simulink model "Demo_PreScanCarSim3D_ExtFMU_cs"  (Simulink 8.6)
settings: Solver=ode5  SolverMode=SingleTasking  StartTime=0.0  StopTime=68  FixedStep=1/1000  RelTol=1e-3
PreLoadFcn:
  | mbxruntime.callbacks.PreLoadFcn(bdroot);
  | check_NUTS_defined;
  | 
  | assignin('base',['model_closed_' bdroot],false);
PostLoadFcn:
  | mbxruntime.callbacks.PostLoadFcn(bdroot);
InitFcn:
  | mbxruntime.callbacks.InitFcn(bdroot);
StartFcn:
  | mbxruntime.callbacks.StartFcn(bdroot);
StopFcn:
  | mbxruntime.callbacks.StopFcn(bdroot);
undefined symbols (not defined in the file): DiscIntNeverNeededParam, mbxruntime, tabledata, warningInitialVelocity, x0, x_ini_VRML, y_ini_VRML, z_ini_VRML
libraries: PreScanSimulinkLibrary x15, simulink_extras x8, simulink x5, PreScanCarSimLibrary x1
(part 4 of 11)

== system Demo_PreScanCarSim3D_ExtFMU_cs/Audi_A8_1/ENABLED/VISUWheelsCarSim_Mux ==
  StateWheels : Inport
  Bus Selector : BusSelector  OutputSignals=PreScanBUS_VehicleDynamics.Wheel.Position.Linear.Pos_FL_Wheel_CoorSys_V[x;y;z][m],PreScanBUS_VehicleDynamics.Wheel.Position.Angualr.Rot_FL_Wheel_CoorSys_V[x;y;z][deg].Angle_Camber_FL_Wheel_CoorSys_V[deg],PreScanBUS_VehicleDynamics.Wheel.Position.Angualr.Rot_FL_Wheel_CoorSys_V[x;y;z][deg].Angle_Rot_FL_Wheel[deg],PreScanBUS_VehicleDynamics.Wheel.Position.Angualr.Rot_FL_Wheel_CoorSys_V[x;y;z][deg].Angle_Toe_FL_Wheel_CoorSys_V[deg],PreScanBUS_VehicleDynamics.Wheel.Position.Linear.Pos_FR_Wheel_CoorSys_V[x;y;z][m],PreScanBUS_VehicleDynamics.Wheel.Position.Angualr.Rot_FR_Wheel_CoorSys_V[x;y;z][deg].Angle_Camber_FR_Wheel_CoorSys_V[deg],PreScanBUS_VehicleDynamics.Wheel.Position.Angualr.Rot_FR_Wheel_CoorSys_V[x;y;z][deg].Angle_Rot_FR_Wheel[deg],PreScanBUS_VehicleDynamics.Wheel.Position.Angualr.Rot_FR_Wheel_CoorSys_V[x;y;z][deg].Angle_Toe_FR_Wheel_CoorSys_V[deg],PreScanBUS_VehicleDynamics.Wheel.Position.Linear.Pos_RL_Wheel_CoorSys_V[x;y;z][m],PreScanBUS_VehicleDynamics.Wheel.Position.Angualr.Rot_RL_Wheel_CoorSys_V[x;y;z][deg].Angle_Camber_RL_Wheel_CoorSys_V[deg],PreScanBUS_VehicleDynamics.Wheel.Position.Angualr.Rot_RL_Wheel_CoorSys_V[x;y;z][deg].Angle_Rot_RL_Wheel[deg],PreScanBUS_VehicleDynamics.Wheel.Position.Angualr.Rot_RL_Wheel_CoorSys_V[x;y;z][deg].Angle_Toe_RL_Wheel_CoorSys_V[deg],PreScanBUS_VehicleDynamics.Wheel.Position.Linear.Pos_RR_Wheel_CoorSys_V[x;y;z][m],PreScanBUS_VehicleDynamics.Wheel.Position.Angualr.Rot_RR_Wheel_CoorSys_V[x;y;z][deg].Angle_Camber_RR_Wheel_CoorSys_V[deg],PreScanBUS_VehicleDynamics.Wheel.Position.Angualr.Rot_RR_Wheel_CoorSys_V[x;y;z][deg].Angle_Rot_RR_Wheel[deg],PreScanBUS_VehicleDynamics.Wheel.Position.Angualr.Rot_RR_Wheel_CoorSys_V[x;y;z][deg].Angle_Toe_RR_Wheel_CoorSys_V[deg]
  Demux{,1..3} (4 alike) : Demux  Outputs=3
  Mux{,1..4,6..8} (8 alike) : Mux  Inputs=3
  Mux5 : Mux  Inputs=[3 3 3 3 3 3 3 3]
  Wheels : Outport
  wires:
  Bus Selector/16 -> Mux3/3  "<Angle_Toe_RR_Wheel_CoorSys_V[deg]>"
  Bus Selector/15 -> Mux3/2  "<Angle_Rot_RR_Wheel[deg]>"
  Bus Selector/14 -> Mux3/1  "<Angle_Camber_RR_Wheel_CoorSys_V[deg]>"
  Bus Selector/13 -> Demux3/1  "<Pos_RR_Wheel_CoorSys_V[x;y;z][m]>"
  Demux3/3 -> Mux8/3
  Demux3/2 -> Mux8/2
  Demux3/1 -> Mux8/1
  Bus Selector/12 -> Mux2/3  "<Angle_Toe_RL_Wheel_CoorSys_V[deg]>"
  Bus Selector/11 -> Mux2/2  "<Angle_Rot_RL_Wheel[deg]>"
  Bus Selector/10 -> Mux2/1  "<Angle_Camber_RL_Wheel_CoorSys_V[deg]>"
  Bus Selector/9 -> Demux2/1  "<Pos_RL_Wheel_CoorSys_V[x;y;z][m]>"
  Demux2/3 -> Mux7/3
  Demux2/2 -> Mux7/2
  Demux2/1 -> Mux7/1
  Bus Selector/8 -> Mux1/3  "<Angle_Toe_FR_Wheel_CoorSys_V[deg]>"
  Bus Selector/7 -> Mux1/2  "<Angle_Rot_FR_Wheel[deg]>"
  Bus Selector/6 -> Mux1/1  "<Angle_Camber_FR_Wheel_CoorSys_V[deg]>"
  Bus Selector/5 -> Demux1/1  "<Pos_FR_Wheel_CoorSys_V[x;y;z][m]>"
  Demux1/3 -> Mux6/3
  Demux1/2 -> Mux6/2
  Demux1/1 -> Mux6/1
  Bus Selector/4 -> Mux/3  "<Angle_Toe_FL_Wheel_CoorSys_V[deg]>"
  Bus Selector/3 -> Mux/2  "<Angle_Rot_FL_Wheel[deg]>"
  Bus Selector/2 -> Mux/1  "<Angle_Camber_FL_Wheel_CoorSys_V[deg]>"
  Demux/3 -> Mux4/3
  Demux/2 -> Mux4/2
  Demux/1 -> Mux4/1
  Bus Selector/1 -> Demux/1  "<Pos_FL_Wheel_CoorSys_V[x;y;z][m]>"
  StateWheels/1 -> Bus Selector/1
  Mux2/1 -> Mux5/6  "xyz rotation RL [deg]"
  Mux3/1 -> Mux5/8  "xyz rotation RR [deg]"
  Mux/1 -> Mux5/2  "xyz rotation FL [deg]"
  Mux1/1 -> Mux5/4  "xyz rotation FR [deg]"
  Mux5/1 -> Wheels/1
  Mux4/1 -> Mux5/1  "xyz displacement FL [m]"
  Mux6/1 -> Mux5/3  "xyz displacement FR [m]"
  Mux8/1 -> Mux5/7  "xyz displacement RR [m]"
  Mux7/1 -> Mux5/5  "xyz displacement RL [m]"

== system Demo_PreScanCarSim3D_ExtFMU_cs/Box_1/DISABLED/GND1 ==
  GND_AccelerationX : Constant  Value=0
  GND_AccelerationY : Constant  Value=0
  GND_AccelerationZ : Constant  Value=0
  GND_AngularVelocityPitch : Constant  Value=0
  GND_AngularVelocityRoll : Constant  Value=0
  GND_AngularVelocityYaw : Constant  Value=0
  GND_OrientationPitch : Constant  Value=0
  GND_OrientationRoll : Constant  Value=0
  GND_OrientationYaw : Constant  Value=0
  GND_PositionX : Constant  Value=0
  GND_PositionY : Constant  Value=0
  GND_PositionZ : Constant  Value=0
  GND_VelocityX : Constant  Value=0
  GND_VelocityY : Constant  Value=0
  GND_VelocityZ : Constant  Value=0
  buscreator : BusCreator  Inputs=15  OutDataTypeStr=Bus: PRESCAN_STATEACTUATORDATA  NonVirtualBus=on
  bus : Outport  OutDataTypeStr=Bus: PRESCAN_STATEACTUATORDATA
  wires:
  GND_PositionX/1 -> buscreator/1  "PositionX"
  GND_PositionY/1 -> buscreator/2  "PositionY"
  GND_PositionZ/1 -> buscreator/3  "PositionZ"
  GND_VelocityX/1 -> buscreator/4  "VelocityX"
  GND_VelocityY/1 -> buscreator/5  "VelocityY"
  GND_VelocityZ/1 -> buscreator/6  "VelocityZ"
  GND_AccelerationX/1 -> buscreator/7  "AccelerationX"
  GND_AccelerationY/1 -> buscreator/8  "AccelerationY"
  GND_AccelerationZ/1 -> buscreator/9  "AccelerationZ"
  GND_OrientationRoll/1 -> buscreator/10  "OrientationRoll"
  GND_OrientationPitch/1 -> buscreator/11  "OrientationPitch"
  GND_OrientationYaw/1 -> buscreator/12  "OrientationYaw"
  GND_AngularVelocityRoll/1 -> buscreator/13  "AngularVelocityRoll"
  GND_AngularVelocityPitch/1 -> buscreator/14  "AngularVelocityPitch"
  GND_AngularVelocityYaw/1 -> buscreator/15  "AngularVelocityYaw"
  buscreator/1 -> bus/1

== system Demo_PreScanCarSim3D_ExtFMU_cs/Box_1/ENABLED/Dynamics_Empty ==
  note: For state mode 'Dynamic' positions
      | are not taken into account, as they
      | are computed by integrating velocity.
      | Click annotation for Help.
  Ground_{1..9} (9 alike) : Ground
  MuxState : Subsystem  Tag=mux/State  mask(Empty Dynamics State Block){positioningmode=on, TimeStep=50/1000}
      mask prompts: positioningmode "Positioning Mode"; TimeStep "Auto Assigned: Time Step [s]"
      mask help:
      | Build the state of an actor based on user input.
      | The user can either use positioning mode or dynamics mode.
      | - When using positioning mode the position and orientation of the actor are set directly based on the input. Expected input is relative to the initial position and orientation of the actor. It's also possible to specify the velocity of the actor, though this input isn't used, only passed on.
      | - When using dynamics mode the position input is ignored. Expected input is velocity and orientation. The velocity is relative the current orientation of the actor, while orientation is relative to its initial orientation. The position of the actor is calculated based on the velocity and orientation given.
      settings: DeleteFcn=PreScanBlockDeleteFcn;
  State : Outport  Tag=outport/StateOutport  SampleTime=50/1000
  wires:
  MuxState/1(state) -> State/1
  Ground_1/1 -> MuxState/1(x [m])
  Ground_2/1 -> MuxState/2(y [m])
  Ground_3/1 -> MuxState/3(z [m])
  Ground_4/1 -> MuxState/4(dx [m/s])
  Ground_5/1 -> MuxState/5(dy [m/s])
  Ground_6/1 -> MuxState/6(dz [m/s])
  Ground_7/1 -> MuxState/7(R [rad])
  Ground_8/1 -> MuxState/8(P [rad])
  Ground_9/1 -> MuxState/9(Y [rad])

== system Demo_PreScanCarSim3D_ExtFMU_cs/Box_1/ENABLED/SELF_Demux ==
  SELF : Inport  OutDataTypeStr=Bus: PRESCAN_SELFSENSORDATA
  Bus Selector : BusSelector  OutputSignals=PositionX,PositionY,PositionZ,OrientationRoll,OrientationPitch,OrientationYaw,Velocity,Yaw_rate,Lat,Long,Alt
  Demux2 : Demux  Outputs=3
  Gain : Gain  Gain=180/pi
  Gain1 : Gain  Gain=180/pi
  Vector Concatenate1 : Concatenate  NumInputs=3
  compas converter : Subsystem
  x [m] : Outport
  y [m] : Outport  Port=2
  z [m] : Outport  Port=3
  rotx [deg] : Outport  Port=4
  roty [deg] : Outport  Port=5
  rotz [deg] : Outport  Port=6
  GPS lat [deg] : Outport  Port=7
  GPS long [deg] : Outport  Port=8
  GPS alt [m] : Outport  Port=9
  velocity [m/s] : Outport  Port=10
  heading [deg] : Outport  Port=11
  yaw rate [deg/s] : Outport  Port=12
  wires:
  Bus Selector/11 -> GPS alt [m]/1  "<Alt>"
  Bus Selector/10 -> GPS long [deg]/1  "<Long>"
  Bus Selector/9 -> GPS lat [deg]/1  "<Lat>"
  Bus Selector/8 -> Gain1/1  "<Yaw_rate>"
  Bus Selector/7 -> velocity [m/s]/1  "<Velocity>"
  Bus Selector/6 -> compas converter/1(rotz [rad]), Vector Concatenate1/3  "<OrientationYaw>"
  Bus Selector/5 -> Vector Concatenate1/2  "<OrientationPitch>"
  Bus Selector/4 -> Vector Concatenate1/1  "<OrientationRoll>"
  Vector Concatenate1/1 -> Gain/1
  Bus Selector/3 -> z [m]/1  "<PositionZ>"
  Bus Selector/2 -> y [m]/1  "<PositionY>"
  Bus Selector/1 -> x [m]/1  "<PositionX>"
  SELF/1 -> Bus Selector/1
  Gain/1 -> Demux2/1
  Demux2/1 -> rotx [deg]/1
  Demux2/2 -> roty [deg]/1
  Demux2/3 -> rotz [deg]/1
  compas converter/1(heading [deg]) -> heading [deg]/1
  Gain1/1 -> yaw rate [deg/s]/1

== system Demo_PreScanCarSim3D_ExtFMU_cs/Box_1/ENABLED/STATE_Box_1 ==
  State : Inport  SampleTime=TimeStep
  Bus Creator : BusCreator  Inputs=15  OutDataTypeStr=Bus: PRESCAN_STATEACTUATORDATA  NonVirtualBus=on
  Demux : Demux  Outputs=15
  iniBODYAngles wrtVEH [rad] : Constant  Value=[Roll0 Pitch0 0]  SampleTime=TimeStep
  iniVEHAngles wrtGLOB [rad] : Constant  Value=[0 0 Yaw0]  SampleTime=TimeStep
  iniVEHposition wrtGLOB [m] : Constant  Value=[x0 y0 z0]  SampleTime=TimeStep
  state2FullState : PreScanSimulinkLibrary/state2FullState  SystemSampleTime=-1
  StateBus : Outport  OutDataTypeStr=Bus: PRESCAN_STATEACTUATORDATA
  wires:
  Bus Creator/1 -> StateBus/1
  State/1 -> state2FullState/1
  state2FullState/1 -> Demux/1
  iniVEHposition wrtGLOB [m]/1 -> state2FullState/2
  iniBODYAngles wrtVEH [rad]/1 -> state2FullState/3
  iniVEHAngles wrtGLOB [rad]/1 -> state2FullState/4
  Demux/1 -> Bus Creator/1  "PositionX"
  Demux/2 -> Bus Creator/2  "PositionY"
  Demux/3 -> Bus Creator/3  "PositionZ"
  Demux/4 -> Bus Creator/4  "VelocityX"
  Demux/5 -> Bus Creator/5  "VelocityY"
  Demux/6 -> Bus Creator/6  "VelocityZ"
  Demux/7 -> Bus Creator/7  "AccelerationX"
  Demux/8 -> Bus Creator/8  "AccelerationY"
  Demux/9 -> Bus Creator/9  "AccelerationZ"
  Demux/10 -> Bus Creator/10  "OrientationRoll"
  Demux/11 -> Bus Creator/11  "OrientationPitch"
  Demux/12 -> Bus Creator/12  "OrientationYaw"
  Demux/13 -> Bus Creator/13  "AngularVelocityRoll"
  Demux/14 -> Bus Creator/14  "AngularVelocityPitch"
  Demux/15 -> Bus Creator/15  "AngularVelocityYaw"

== system Demo_PreScanCarSim3D_ExtFMU_cs/Box_2/DISABLED/GND1 ==
  GND_AccelerationX : Constant  Value=0
  GND_AccelerationY : Constant  Value=0
  GND_AccelerationZ : Constant  Value=0
  GND_AngularVelocityPitch : Constant  Value=0
  GND_AngularVelocityRoll : Constant  Value=0
  GND_AngularVelocityYaw : Constant  Value=0
  GND_OrientationPitch : Constant  Value=0
  GND_OrientationRoll : Constant  Value=0
  GND_OrientationYaw : Constant  Value=0
  GND_PositionX : Constant  Value=0
  GND_PositionY : Constant  Value=0
  GND_PositionZ : Constant  Value=0
  GND_VelocityX : Constant  Value=0
  GND_VelocityY : Constant  Value=0
  GND_VelocityZ : Constant  Value=0
  buscreator : BusCreator  Inputs=15  OutDataTypeStr=Bus: PRESCAN_STATEACTUATORDATA  NonVirtualBus=on
  bus : Outport  OutDataTypeStr=Bus: PRESCAN_STATEACTUATORDATA
  wires:
  GND_PositionX/1 -> buscreator/1  "PositionX"
  GND_PositionY/1 -> buscreator/2  "PositionY"
  GND_PositionZ/1 -> buscreator/3  "PositionZ"
  GND_VelocityX/1 -> buscreator/4  "VelocityX"
  GND_VelocityY/1 -> buscreator/5  "VelocityY"
  GND_VelocityZ/1 -> buscreator/6  "VelocityZ"
  GND_AccelerationX/1 -> buscreator/7  "AccelerationX"
  GND_AccelerationY/1 -> buscreator/8  "AccelerationY"
  GND_AccelerationZ/1 -> buscreator/9  "AccelerationZ"
  GND_OrientationRoll/1 -> buscreator/10  "OrientationRoll"
  GND_OrientationPitch/1 -> buscreator/11  "OrientationPitch"
  GND_OrientationYaw/1 -> buscreator/12  "OrientationYaw"
  GND_AngularVelocityRoll/1 -> buscreator/13  "AngularVelocityRoll"
  GND_AngularVelocityPitch/1 -> buscreator/14  "AngularVelocityPitch"
  GND_AngularVelocityYaw/1 -> buscreator/15  "AngularVelocityYaw"
  buscreator/1 -> bus/1

== system Demo_PreScanCarSim3D_ExtFMU_cs/Box_2/ENABLED/Dynamics_Empty ==
  note: For state mode 'Dynamic' positions
      | are not taken into account, as they
      | are computed by integrating velocity.
      | Click annotation for Help.
  Ground_{1..9} (9 alike) : Ground
  MuxState : Subsystem  Tag=mux/State  mask(Empty Dynamics State Block){positioningmode=on, TimeStep=50/1000}
      mask prompts: positioningmode "Positioning Mode"; TimeStep "Auto Assigned: Time Step [s]"
      mask help:
      | Build the state of an actor based on user input.
      | The user can either use positioning mode or dynamics mode.
      | - When using positioning mode the position and orientation of the actor are set directly based on the input. Expected input is relative to the initial position and orientation of the actor. It's also possible to specify the velocity of the actor, though this input isn't used, only passed on.
      | - When using dynamics mode the position input is ignored. Expected input is velocity and orientation. The velocity is relative the current orientation of the actor, while orientation is relative to its initial orientation. The position of the actor is calculated based on the velocity and orientation given.
      settings: DeleteFcn=PreScanBlockDeleteFcn;
  State : Outport  Tag=outport/StateOutport  SampleTime=50/1000
  wires:
  MuxState/1(state) -> State/1
  Ground_1/1 -> MuxState/1(x [m])
  Ground_2/1 -> MuxState/2(y [m])
  Ground_3/1 -> MuxState/3(z [m])
  Ground_4/1 -> MuxState/4(dx [m/s])
  Ground_5/1 -> MuxState/5(dy [m/s])
  Ground_6/1 -> MuxState/6(dz [m/s])
  Ground_7/1 -> MuxState/7(R [rad])
  Ground_8/1 -> MuxState/8(P [rad])
  Ground_9/1 -> MuxState/9(Y [rad])

== system Demo_PreScanCarSim3D_ExtFMU_cs/Box_2/ENABLED/SELF_Demux ==
  SELF : Inport  OutDataTypeStr=Bus: PRESCAN_SELFSENSORDATA
  Bus Selector : BusSelector  OutputSignals=PositionX,PositionY,PositionZ,OrientationRoll,OrientationPitch,OrientationYaw,Velocity,Yaw_rate,Lat,Long,Alt
  Demux2 : Demux  Outputs=3
  Gain : Gain  Gain=180/pi
  Gain1 : Gain  Gain=180/pi
  Vector Concatenate1 : Concatenate  NumInputs=3
  compas converter : Subsystem
  x [m] : Outport
  y [m] : Outport  Port=2
  z [m] : Outport  Port=3
  rotx [deg] : Outport  Port=4
  roty [deg] : Outport  Port=5
  rotz [deg] : Outport  Port=6
  GPS lat [deg] : Outport  Port=7
  GPS long [deg] : Outport  Port=8
  GPS alt [m] : Outport  Port=9
  velocity [m/s] : Outport  Port=10
  heading [deg] : Outport  Port=11
  yaw rate [deg/s] : Outport  Port=12
  wires:
  Bus Selector/11 -> GPS alt [m]/1  "<Alt>"
  Bus Selector/10 -> GPS long [deg]/1  "<Long>"
  Bus Selector/9 -> GPS lat [deg]/1  "<Lat>"
  Bus Selector/8 -> Gain1/1  "<Yaw_rate>"
  Bus Selector/7 -> velocity [m/s]/1  "<Velocity>"
  Bus Selector/6 -> compas converter/1(rotz [rad]), Vector Concatenate1/3  "<OrientationYaw>"
  Bus Selector/5 -> Vector Concatenate1/2  "<OrientationPitch>"
  Bus Selector/4 -> Vector Concatenate1/1  "<OrientationRoll>"
  Vector Concatenate1/1 -> Gain/1
  Bus Selector/3 -> z [m]/1  "<PositionZ>"
  Bus Selector/2 -> y [m]/1  "<PositionY>"
  Bus Selector/1 -> x [m]/1  "<PositionX>"
  SELF/1 -> Bus Selector/1
  Gain/1 -> Demux2/1
  Demux2/1 -> rotx [deg]/1
  Demux2/2 -> roty [deg]/1
  Demux2/3 -> rotz [deg]/1
  compas converter/1(heading [deg]) -> heading [deg]/1
  Gain1/1 -> yaw rate [deg/s]/1

== system Demo_PreScanCarSim3D_ExtFMU_cs/Box_2/ENABLED/STATE_Box_2 ==
  State : Inport  SampleTime=TimeStep
  Bus Creator : BusCreator  Inputs=15  OutDataTypeStr=Bus: PRESCAN_STATEACTUATORDATA  NonVirtualBus=on
  Demux : Demux  Outputs=15
  iniBODYAngles wrtVEH [rad] : Constant  Value=[Roll0 Pitch0 0]  SampleTime=TimeStep
  iniVEHAngles wrtGLOB [rad] : Constant  Value=[0 0 Yaw0]  SampleTime=TimeStep
  iniVEHposition wrtGLOB [m] : Constant  Value=[x0 y0 z0]  SampleTime=TimeStep
  state2FullState : PreScanSimulinkLibrary/state2FullState  SystemSampleTime=-1
  StateBus : Outport  OutDataTypeStr=Bus: PRESCAN_STATEACTUATORDATA
  wires:
  Bus Creator/1 -> StateBus/1
  State/1 -> state2FullState/1
  state2FullState/1 -> Demux/1
  iniVEHposition wrtGLOB [m]/1 -> state2FullState/2
  iniBODYAngles wrtVEH [rad]/1 -> state2FullState/3
  iniVEHAngles wrtGLOB [rad]/1 -> state2FullState/4
  Demux/1 -> Bus Creator/1  "PositionX"
  Demux/2 -> Bus Creator/2  "PositionY"
  Demux/3 -> Bus Creator/3  "PositionZ"
  Demux/4 -> Bus Creator/4  "VelocityX"
  Demux/5 -> Bus Creator/5  "VelocityY"
  Demux/6 -> Bus Creator/6  "VelocityZ"
  Demux/7 -> Bus Creator/7  "AccelerationX"
  Demux/8 -> Bus Creator/8  "AccelerationY"
  Demux/9 -> Bus Creator/9  "AccelerationZ"
  Demux/10 -> Bus Creator/10  "OrientationRoll"
  Demux/11 -> Bus Creator/11  "OrientationPitch"
  Demux/12 -> Bus Creator/12  "OrientationYaw"
  Demux/13 -> Bus Creator/13  "AngularVelocityRoll"
  Demux/14 -> Bus Creator/14  "AngularVelocityPitch"
  Demux/15 -> Bus Creator/15  "AngularVelocityYaw"

== system Demo_PreScanCarSim3D_ExtFMU_cs/Box_3/DISABLED/GND1 ==
  GND_AccelerationX : Constant  Value=0
  GND_AccelerationY : Constant  Value=0
  GND_AccelerationZ : Constant  Value=0
  GND_AngularVelocityPitch : Constant  Value=0
  GND_AngularVelocityRoll : Constant  Value=0
  GND_AngularVelocityYaw : Constant  Value=0
  GND_OrientationPitch : Constant  Value=0
  GND_OrientationRoll : Constant  Value=0
  GND_OrientationYaw : Constant  Value=0
  GND_PositionX : Constant  Value=0
  GND_PositionY : Constant  Value=0
  GND_PositionZ : Constant  Value=0
  GND_VelocityX : Constant  Value=0
  GND_VelocityY : Constant  Value=0
  GND_VelocityZ : Constant  Value=0
  buscreator : BusCreator  Inputs=15  OutDataTypeStr=Bus: PRESCAN_STATEACTUATORDATA  NonVirtualBus=on
  bus : Outport  OutDataTypeStr=Bus: PRESCAN_STATEACTUATORDATA
  wires:
  GND_PositionX/1 -> buscreator/1  "PositionX"
  GND_PositionY/1 -> buscreator/2  "PositionY"
  GND_PositionZ/1 -> buscreator/3  "PositionZ"
  GND_VelocityX/1 -> buscreator/4  "VelocityX"
  GND_VelocityY/1 -> buscreator/5  "VelocityY"
  GND_VelocityZ/1 -> buscreator/6  "VelocityZ"
  GND_AccelerationX/1 -> buscreator/7  "AccelerationX"
  GND_AccelerationY/1 -> buscreator/8  "AccelerationY"
  GND_AccelerationZ/1 -> buscreator/9  "AccelerationZ"
  GND_OrientationRoll/1 -> buscreator/10  "OrientationRoll"
  GND_OrientationPitch/1 -> buscreator/11  "OrientationPitch"
  GND_OrientationYaw/1 -> buscreator/12  "OrientationYaw"
  GND_AngularVelocityRoll/1 -> buscreator/13  "AngularVelocityRoll"
  GND_AngularVelocityPitch/1 -> buscreator/14  "AngularVelocityPitch"
  GND_AngularVelocityYaw/1 -> buscreator/15  "AngularVelocityYaw"
  buscreator/1 -> bus/1

== system Demo_PreScanCarSim3D_ExtFMU_cs/Box_3/ENABLED/Dynamics_Empty ==
  note: For state mode 'Dynamic' positions
      | are not taken into account, as they
      | are computed by integrating velocity.
      | Click annotation for Help.
  Ground_{1..9} (9 alike) : Ground
  MuxState : Subsystem  Tag=mux/State  mask(Empty Dynamics State Block){positioningmode=on, TimeStep=50/1000}
      mask prompts: positioningmode "Positioning Mode"; TimeStep "Auto Assigned: Time Step [s]"
      mask help:
      | Build the state of an actor based on user input.
      | The user can either use positioning mode or dynamics mode.
      | - When using positioning mode the position and orientation of the actor are set directly based on the input. Expected input is relative to the initial position and orientation of the actor. It's also possible to specify the velocity of the actor, though this input isn't used, only passed on.
      | - When using dynamics mode the position input is ignored. Expected input is velocity and orientation. The velocity is relative the current orientation of the actor, while orientation is relative to its initial orientation. The position of the actor is calculated based on the velocity and orientation given.
      settings: DeleteFcn=PreScanBlockDeleteFcn;
  State : Outport  Tag=outport/StateOutport  SampleTime=50/1000
  wires:
  MuxState/1(state) -> State/1
  Ground_1/1 -> MuxState/1(x [m])
  Ground_2/1 -> MuxState/2(y [m])
  Ground_3/1 -> MuxState/3(z [m])
  Ground_4/1 -> MuxState/4(dx [m/s])
  Ground_5/1 -> MuxState/5(dy [m/s])
  Ground_6/1 -> MuxState/6(dz [m/s])
  Ground_7/1 -> MuxState/7(R [rad])
  Ground_8/1 -> MuxState/8(P [rad])
  Ground_9/1 -> MuxState/9(Y [rad])

== system Demo_PreScanCarSim3D_ExtFMU_cs/Box_3/ENABLED/SELF_Demux ==
  SELF : Inport  OutDataTypeStr=Bus: PRESCAN_SELFSENSORDATA
  Bus Selector : BusSelector  OutputSignals=PositionX,PositionY,PositionZ,OrientationRoll,OrientationPitch,OrientationYaw,Velocity,Yaw_rate,Lat,Long,Alt
  Demux2 : Demux  Outputs=3
  Gain : Gain  Gain=180/pi
  Gain1 : Gain  Gain=180/pi
  Vector Concatenate1 : Concatenate  NumInputs=3
  compas converter : Subsystem
  x [m] : Outport
  y [m] : Outport  Port=2
  z [m] : Outport  Port=3
  rotx [deg] : Outport  Port=4
  roty [deg] : Outport  Port=5
  rotz [deg] : Outport  Port=6
  GPS lat [deg] : Outport  Port=7
  GPS long [deg] : Outport  Port=8
  GPS alt [m] : Outport  Port=9
  velocity [m/s] : Outport  Port=10
  heading [deg] : Outport  Port=11
  yaw rate [deg/s] : Outport  Port=12
  wires:
  Bus Selector/11 -> GPS alt [m]/1  "<Alt>"
  Bus Selector/10 -> GPS long [deg]/1  "<Long>"
  Bus Selector/9 -> GPS lat [deg]/1  "<Lat>"
  Bus Selector/8 -> Gain1/1  "<Yaw_rate>"
  Bus Selector/7 -> velocity [m/s]/1  "<Velocity>"
  Bus Selector/6 -> compas converter/1(rotz [rad]), Vector Concatenate1/3  "<OrientationYaw>"
  Bus Selector/5 -> Vector Concatenate1/2  "<OrientationPitch>"
  Bus Selector/4 -> Vector Concatenate1/1  "<OrientationRoll>"
  Vector Concatenate1/1 -> Gain/1
  Bus Selector/3 -> z [m]/1  "<PositionZ>"
  Bus Selector/2 -> y [m]/1  "<PositionY>"
  Bus Selector/1 -> x [m]/1  "<PositionX>"
  SELF/1 -> Bus Selector/1
  Gain/1 -> Demux2/1
  Demux2/1 -> rotx [deg]/1
  Demux2/2 -> roty [deg]/1
  Demux2/3 -> rotz [deg]/1
  compas converter/1(heading [deg]) -> heading [deg]/1
  Gain1/1 -> yaw rate [deg/s]/1

== system Demo_PreScanCarSim3D_ExtFMU_cs/Box_3/ENABLED/STATE_Box_3 ==
  State : Inport  SampleTime=TimeStep
  Bus Creator : BusCreator  Inputs=15  OutDataTypeStr=Bus: PRESCAN_STATEACTUATORDATA  NonVirtualBus=on
  Demux : Demux  Outputs=15
  iniBODYAngles wrtVEH [rad] : Constant  Value=[Roll0 Pitch0 0]  SampleTime=TimeStep
  iniVEHAngles wrtGLOB [rad] : Constant  Value=[0 0 Yaw0]  SampleTime=TimeStep
  iniVEHposition wrtGLOB [m] : Constant  Value=[x0 y0 z0]  SampleTime=TimeStep
  state2FullState : PreScanSimulinkLibrary/state2FullState  SystemSampleTime=-1
  StateBus : Outport  OutDataTypeStr=Bus: PRESCAN_STATEACTUATORDATA
  wires:
  Bus Creator/1 -> StateBus/1
  State/1 -> state2FullState/1
  state2FullState/1 -> Demux/1
  iniVEHposition wrtGLOB [m]/1 -> state2FullState/2
  iniBODYAngles wrtVEH [rad]/1 -> state2FullState/3
  iniVEHAngles wrtGLOB [rad]/1 -> state2FullState/4
  Demux/1 -> Bus Creator/1  "PositionX"
  Demux/2 -> Bus Creator/2  "PositionY"
  Demux/3 -> Bus Creator/3  "PositionZ"
  Demux/4 -> Bus Creator/4  "VelocityX"
  Demux/5 -> Bus Creator/5  "VelocityY"
  Demux/6 -> Bus Creator/6  "VelocityZ"
  Demux/7 -> Bus Creator/7  "AccelerationX"
  Demux/8 -> Bus Creator/8  "AccelerationY"
  Demux/9 -> Bus Creator/9  "AccelerationZ"
  Demux/10 -> Bus Creator/10  "OrientationRoll"
  Demux/11 -> Bus Creator/11  "OrientationPitch"
  Demux/12 -> Bus Creator/12  "OrientationYaw"
  Demux/13 -> Bus Creator/13  "AngularVelocityRoll"
  Demux/14 -> Bus Creator/14  "AngularVelocityPitch"
  Demux/15 -> Bus Creator/15  "AngularVelocityYaw"

== system Demo_PreScanCarSim3D_ExtFMU_cs/Box_4/DISABLED/GND1 ==
  GND_AccelerationX : Constant  Value=0
  GND_AccelerationY : Constant  Value=0
  GND_AccelerationZ : Constant  Value=0
  GND_AngularVelocityPitch : Constant  Value=0
  GND_AngularVelocityRoll : Constant  Value=0
  GND_AngularVelocityYaw : Constant  Value=0
  GND_OrientationPitch : Constant  Value=0
  GND_OrientationRoll : Constant  Value=0
  GND_OrientationYaw : Constant  Value=0
  GND_PositionX : Constant  Value=0
  GND_PositionY : Constant  Value=0
  GND_PositionZ : Constant  Value=0
  GND_VelocityX : Constant  Value=0
  GND_VelocityY : Constant  Value=0
  GND_VelocityZ : Constant  Value=0
  buscreator : BusCreator  Inputs=15  OutDataTypeStr=Bus: PRESCAN_STATEACTUATORDATA  NonVirtualBus=on
  bus : Outport  OutDataTypeStr=Bus: PRESCAN_STATEACTUATORDATA
  wires:
  GND_PositionX/1 -> buscreator/1  "PositionX"
  GND_PositionY/1 -> buscreator/2  "PositionY"
  GND_PositionZ/1 -> buscreator/3  "PositionZ"
  GND_VelocityX/1 -> buscreator/4  "VelocityX"
  GND_VelocityY/1 -> buscreator/5  "VelocityY"
  GND_VelocityZ/1 -> buscreator/6  "VelocityZ"
  GND_AccelerationX/1 -> buscreator/7  "AccelerationX"
  GND_AccelerationY/1 -> buscreator/8  "AccelerationY"
  GND_AccelerationZ/1 -> buscreator/9  "AccelerationZ"
  GND_OrientationRoll/1 -> buscreator/10  "OrientationRoll"
  GND_OrientationPitch/1 -> buscreator/11  "OrientationPitch"
  GND_OrientationYaw/1 -> buscreator/12  "OrientationYaw"
  GND_AngularVelocityRoll/1 -> buscreator/13  "AngularVelocityRoll"
  GND_AngularVelocityPitch/1 -> buscreator/14  "AngularVelocityPitch"
  GND_AngularVelocityYaw/1 -> buscreator/15  "AngularVelocityYaw"
  buscreator/1 -> bus/1

== system Demo_PreScanCarSim3D_ExtFMU_cs/Box_4/ENABLED/Dynamics_Empty ==
  note: For state mode 'Dynamic' positions
      | are not taken into account, as they
      | are computed by integrating velocity.
      | Click annotation for Help.
  Ground_{1..9} (9 alike) : Ground
  MuxState : Subsystem  Tag=mux/State  mask(Empty Dynamics State Block){positioningmode=on, TimeStep=50/1000}
      mask prompts: positioningmode "Positioning Mode"; TimeStep "Auto Assigned: Time Step [s]"
      mask help:
      | Build the state of an actor based on user input.
      | The user can either use positioning mode or dynamics mode.
      | - When using positioning mode the position and orientation of the actor are set directly based on the input. Expected input is relative to the initial position and orientation of the actor. It's also possible to specify the velocity of the actor, though this input isn't used, only passed on.
      | - When using dynamics mode the position input is ignored. Expected input is velocity and orientation. The velocity is relative the current orientation of the actor, while orientation is relative to its initial orientation. The position of the actor is calculated based on the velocity and orientation given.
      settings: DeleteFcn=PreScanBlockDeleteFcn;
  State : Outport  Tag=outport/StateOutport  SampleTime=50/1000
  wires:
  MuxState/1(state) -> State/1
  Ground_1/1 -> MuxState/1(x [m])
  Ground_2/1 -> MuxState/2(y [m])
  Ground_3/1 -> MuxState/3(z [m])
  Ground_4/1 -> MuxState/4(dx [m/s])
  Ground_5/1 -> MuxState/5(dy [m/s])
  Ground_6/1 -> MuxState/6(dz [m/s])
  Ground_7/1 -> MuxState/7(R [rad])
  Ground_8/1 -> MuxState/8(P [rad])
  Ground_9/1 -> MuxState/9(Y [rad])

== system Demo_PreScanCarSim3D_ExtFMU_cs/Box_4/ENABLED/SELF_Demux ==
  SELF : Inport  OutDataTypeStr=Bus: PRESCAN_SELFSENSORDATA
  Bus Selector : BusSelector  OutputSignals=PositionX,PositionY,PositionZ,OrientationRoll,OrientationPitch,OrientationYaw,Velocity,Yaw_rate,Lat,Long,Alt
  Demux2 : Demux  Outputs=3
  Gain : Gain  Gain=180/pi
  Gain1 : Gain  Gain=180/pi
  Vector Concatenate1 : Concatenate  NumInputs=3
  compas converter : Subsystem
  x [m] : Outport
  y [m] : Outport  Port=2
  z [m] : Outport  Port=3
  rotx [deg] : Outport  Port=4
  roty [deg] : Outport  Port=5
  rotz [deg] : Outport  Port=6
  GPS lat [deg] : Outport  Port=7
  GPS long [deg] : Outport  Port=8
  GPS alt [m] : Outport  Port=9
  velocity [m/s] : Outport  Port=10
  heading [deg] : Outport  Port=11
  yaw rate [deg/s] : Outport  Port=12
  wires:
  Bus Selector/11 -> GPS alt [m]/1  "<Alt>"
  Bus Selector/10 -> GPS long [deg]/1  "<Long>"
  Bus Selector/9 -> GPS lat [deg]/1  "<Lat>"
  Bus Selector/8 -> Gain1/1  "<Yaw_rate>"
  Bus Selector/7 -> velocity [m/s]/1  "<Velocity>"
  Bus Selector/6 -> compas converter/1(rotz [rad]), Vector Concatenate1/3  "<OrientationYaw>"
  Bus Selector/5 -> Vector Concatenate1/2  "<OrientationPitch>"
  Bus Selector/4 -> Vector Concatenate1/1  "<OrientationRoll>"
  Vector Concatenate1/1 -> Gain/1
  Bus Selector/3 -> z [m]/1  "<PositionZ>"
  Bus Selector/2 -> y [m]/1  "<PositionY>"
  Bus Selector/1 -> x [m]/1  "<PositionX>"
  SELF/1 -> Bus Selector/1
  Gain/1 -> Demux2/1
  Demux2/1 -> rotx [deg]/1
  Demux2/2 -> roty [deg]/1
  Demux2/3 -> rotz [deg]/1
  compas converter/1(heading [deg]) -> heading [deg]/1
  Gain1/1 -> yaw rate [deg/s]/1

== system Demo_PreScanCarSim3D_ExtFMU_cs/Box_4/ENABLED/STATE_Box_4 ==
  State : Inport  SampleTime=TimeStep
  Bus Creator : BusCreator  Inputs=15  OutDataTypeStr=Bus: PRESCAN_STATEACTUATORDATA  NonVirtualBus=on
  Demux : Demux  Outputs=15
  iniBODYAngles wrtVEH [rad] : Constant  Value=[Roll0 Pitch0 0]  SampleTime=TimeStep
  iniVEHAngles wrtGLOB [rad] : Constant  Value=[0 0 Yaw0]  SampleTime=TimeStep
  iniVEHposition wrtGLOB [m] : Constant  Value=[x0 y0 z0]  SampleTime=TimeStep
  state2FullState : PreScanSimulinkLibrary/state2FullState  SystemSampleTime=-1
  StateBus : Outport  OutDataTypeStr=Bus: PRESCAN_STATEACTUATORDATA
  wires:
  Bus Creator/1 -> StateBus/1
  State/1 -> state2FullState/1
  state2FullState/1 -> Demux/1
  iniVEHposition wrtGLOB [m]/1 -> state2FullState/2
  iniBODYAngles wrtVEH [rad]/1 -> state2FullState/3
  iniVEHAngles wrtGLOB [rad]/1 -> state2FullState/4
  Demux/1 -> Bus Creator/1  "PositionX"
  Demux/2 -> Bus Creator/2  "PositionY"
  Demux/3 -> Bus Creator/3  "PositionZ"
  Demux/4 -> Bus Creator/4  "VelocityX"
  Demux/5 -> Bus Creator/5  "VelocityY"
  Demux/6 -> Bus Creator/6  "VelocityZ"
  Demux/7 -> Bus Creator/7  "AccelerationX"
  Demux/8 -> Bus Creator/8  "AccelerationY"
  Demux/9 -> Bus Creator/9  "AccelerationZ"
  Demux/10 -> Bus Creator/10  "OrientationRoll"
  Demux/11 -> Bus Creator/11  "OrientationPitch"
  Demux/12 -> Bus Creator/12  "OrientationYaw"
  Demux/13 -> Bus Creator/13  "AngularVelocityRoll"
  Demux/14 -> Bus Creator/14  "AngularVelocityPitch"
  Demux/15 -> Bus Creator/15  "AngularVelocityYaw"

== system Demo_PreScanCarSim3D_ExtFMU_cs/HighwayOverhang_1/ENABLED/VISUMatrixSignLights_Mux ==
  MatrixSign_1 : Inport  Tag=inport/MatrixSign_1  PortDimensions=4  SampleTime=50/1000  BusOutputAsStruct=on
  MatrixSign_2 : Inport  Tag=inport/MatrixSign_2  Port=2  PortDimensions=4  SampleTime=50/1000  BusOutputAsStruct=on
  MatrixSign_3 : Inport  Tag=inport/MatrixSign_3  Port=3  PortDimensions=4  SampleTime=50/1000  BusOutputAsStruct=on
  MatrixSign_4 : Inport  Tag=inport/MatrixSign_4  Port=4  PortDimensions=4  SampleTime=50/1000  BusOutputAsStruct=on
  MuxVisuLights : Mux
  VISUMatrixSignLights_HighwayOverhang_1 : Outport  Tag=outport/VisuMatrixSignLights  SampleTime=50/1000
  wires:
  MuxVisuLights/1 -> VISUMatrixSignLights_HighwayOverhang_1/1
  MatrixSign_1/1 -> MuxVisuLights/1
  MatrixSign_2/1 -> MuxVisuLights/2
  MatrixSign_3/1 -> MuxVisuLights/3
  MatrixSign_4/1 -> MuxVisuLights/4

== system Demo_PreScanCarSim3D_ExtFMU_cs/HighwayOverhang_1/ENABLED/VISUMatrixSign_Mux ==
  MatrixSign_1 : Inport
  MatrixSign_2 : Inport  Port=2
  MatrixSign_3 : Inport  Port=3
  MatrixSign_4 : Inport  Port=4
  MatrixSign_1_Conversion : DataTypeConversion
  MatrixSign_1_InitialResource : Constant  Value=6
  MatrixSign_1_Switch : Switch  Criteria=u2 ~= 0
  MatrixSign_2_Conversion : DataTypeConversion
  MatrixSign_2_InitialResource : Constant  Value=5
  MatrixSign_2_Switch : Switch  Criteria=u2 ~= 0
  MatrixSign_3_Conversion : DataTypeConversion
  MatrixSign_3_InitialResource : Constant  Value=5
  MatrixSign_3_Switch : Switch  Criteria=u2 ~= 0
  MatrixSign_4_Conversion : DataTypeConversion
  MatrixSign_4_InitialResource : Constant  Value=5
  MatrixSign_4_Switch : Switch  Criteria=u2 ~= 0
  SubMuxMatrixSign : Mux
  MatrixSigns : Outport
  wires:
  SubMuxMatrixSign/1 -> MatrixSigns/1
  MatrixSign_1/1 -> MatrixSign_1_Switch/1, MatrixSign_1_Switch/2
  MatrixSign_1_InitialResource/1 -> MatrixSign_1_Switch/3
  MatrixSign_1_Switch/1 -> MatrixSign_1_Conversion/1
  MatrixSign_1_Conversion/1 -> SubMuxMatrixSign/1
  MatrixSign_2/1 -> MatrixSign_2_Switch/1, MatrixSign_2_Switch/2
  MatrixSign_2_InitialResource/1 -> MatrixSign_2_Switch/3
  MatrixSign_2_Switch/1 -> MatrixSign_2_Conversion/1
  MatrixSign_2_Conversion/1 -> SubMuxMatrixSign/2
  MatrixSign_3/1 -> MatrixSign_3_Switch/1, MatrixSign_3_Switch/2
  MatrixSign_3_InitialResource/1 -> MatrixSign_3_Switch/3
  MatrixSign_3_Switch/1 -> MatrixSign_3_Conversion/1
  MatrixSign_3_Conversion/1 -> SubMuxMatrixSign/3
  MatrixSign_4/1 -> MatrixSign_4_Switch/1, MatrixSign_4_Switch/2
  MatrixSign_4_InitialResource/1 -> MatrixSign_4_Switch/3
  MatrixSign_4_Switch/1 -> MatrixSign_4_Conversion/1
  MatrixSign_4_Conversion/1 -> SubMuxMatrixSign/4

== system Demo_PreScanCarSim3D_ExtFMU_cs/HighwayOverhang_2/ENABLED/VISUMatrixSignLights_Mux ==
  MatrixSign_5 : Inport  Tag=inport/MatrixSign_5  PortDimensions=4  SampleTime=50/1000  BusOutputAsStruct=on
  MatrixSign_6 : Inport  Tag=inport/MatrixSign_6  Port=2  PortDimensions=4  SampleTime=50/1000  BusOutputAsStruct=on
  MatrixSign_7 : Inport  Tag=inport/MatrixSign_7  Port=3  PortDimensions=4  SampleTime=50/1000  BusOutputAsStruct=on
  MuxVisuLights : Mux  Inputs=3
  VISUMatrixSignLights_HighwayOverhang_2 : Outport  Tag=outport/VisuMatrixSignLights  SampleTime=50/1000
  wires:
  MuxVisuLights/1 -> VISUMatrixSignLights_HighwayOverhang_2/1
  MatrixSign_5/1 -> MuxVisuLights/1
  MatrixSign_6/1 -> MuxVisuLights/2
  MatrixSign_7/1 -> MuxVisuLights/3

== system Demo_PreScanCarSim3D_ExtFMU_cs/HighwayOverhang_2/ENABLED/VISUMatrixSign_Mux ==
  MatrixSign_5 : Inport
  MatrixSign_6 : Inport  Port=2
  MatrixSign_7 : Inport  Port=3
  MatrixSign_5_Conversion : DataTypeConversion
  MatrixSign_5_InitialResource : Constant  Value=5
  MatrixSign_5_Switch : Switch  Criteria=u2 ~= 0
  MatrixSign_6_Conversion : DataTypeConversion
  MatrixSign_6_InitialResource : Constant  Value=5
  MatrixSign_6_Switch : Switch  Criteria=u2 ~= 0
  MatrixSign_7_Conversion : DataTypeConversion
  MatrixSign_7_InitialResource : Constant  Value=5
  MatrixSign_7_Switch : Switch  Criteria=u2 ~= 0
  SubMuxMatrixSign : Mux  Inputs=3
  MatrixSigns : Outport
  wires:
  SubMuxMatrixSign/1 -> MatrixSigns/1
  MatrixSign_5/1 -> MatrixSign_5_Switch/1, MatrixSign_5_Switch/2
  MatrixSign_5_InitialResource/1 -> MatrixSign_5_Switch/3
  MatrixSign_5_Switch/1 -> MatrixSign_5_Conversion/1
  MatrixSign_5_Conversion/1 -> SubMuxMatrixSign/1
  MatrixSign_6/1 -> MatrixSign_6_Switch/1, MatrixSign_6_Switch/2
  MatrixSign_6_InitialResource/1 -> MatrixSign_6_Switch/3
  MatrixSign_6_Switch/1 -> MatrixSign_6_Conversion/1
  MatrixSign_6_Conversion/1 -> SubMuxMatrixSign/2
  MatrixSign_7/1 -> MatrixSign_7_Switch/1, MatrixSign_7_Switch/2
  MatrixSign_7_InitialResource/1 -> MatrixSign_7_Switch/3
  MatrixSign_7_Switch/1 -> MatrixSign_7_Conversion/1
  MatrixSign_7_Conversion/1 -> SubMuxMatrixSign/3

== system Demo_PreScanCarSim3D_ExtFMU_cs/HighwayOverhang_3/ENABLED/VISUMatrixSignLights_Mux ==
  MatrixSign_10 : Inport  Tag=inport/MatrixSign_10  PortDimensions=4  SampleTime=50/1000  BusOutputAsStruct=on
  MatrixSign_11 : Inport  Tag=inport/MatrixSign_11  Port=2  PortDimensions=4  SampleTime=50/1000  BusOutputAsStruct=on
  MatrixSign_12 : Inport  Tag=inport/MatrixSign_12  Port=3  PortDimensions=4  SampleTime=50/1000  BusOutputAsStruct=on
  MuxVisuLights : Mux  Inputs=3
  VISUMatrixSignLights_HighwayOverhang_3 : Outport  Tag=outport/VisuMatrixSignLights  SampleTime=50/1000
  wires:
  MuxVisuLights/1 -> VISUMatrixSignLights_HighwayOverhang_3/1
  MatrixSign_10/1 -> MuxVisuLights/1
  MatrixSign_11/1 -> MuxVisuLights/2
  MatrixSign_12/1 -> MuxVisuLights/3

== system Demo_PreScanCarSim3D_ExtFMU_cs/HighwayOverhang_3/ENABLED/VISUMatrixSign_Mux ==
  MatrixSign_10 : Inport
  MatrixSign_11 : Inport  Port=2
  MatrixSign_12 : Inport  Port=3
  MatrixSign_10_Conversion : DataTypeConversion
  MatrixSign_10_InitialResource : Constant  Value=9
  MatrixSign_10_Switch : Switch  Criteria=u2 ~= 0
  MatrixSign_11_Conversion : DataTypeConversion
  MatrixSign_11_InitialResource : Constant  Value=9
  MatrixSign_11_Switch : Switch  Criteria=u2 ~= 0
  MatrixSign_12_Conversion : DataTypeConversion
  MatrixSign_12_InitialResource : Constant  Value=9
  MatrixSign_12_Switch : Switch  Criteria=u2 ~= 0
  SubMuxMatrixSign : Mux  Inputs=3
  MatrixSigns : Outport
  wires:
  SubMuxMatrixSign/1 -> MatrixSigns/1
  MatrixSign_10/1 -> MatrixSign_10_Switch/1, MatrixSign_10_Switch/2
  MatrixSign_10_InitialResource/1 -> MatrixSign_10_Switch/3
  MatrixSign_10_Switch/1 -> MatrixSign_10_Conversion/1
  MatrixSign_10_Conversion/1 -> SubMuxMatrixSign/1
  MatrixSign_11/1 -> MatrixSign_11_Switch/1, MatrixSign_11_Switch/2
  MatrixSign_11_InitialResource/1 -> MatrixSign_11_Switch/3
  MatrixSign_11_Switch/1 -> MatrixSign_11_Conversion/1
  MatrixSign_11_Conversion/1 -> SubMuxMatrixSign/2
  MatrixSign_12/1 -> MatrixSign_12_Switch/1, MatrixSign_12_Switch/2
  MatrixSign_12_InitialResource/1 -> MatrixSign_12_Switch/3
  MatrixSign_12_Switch/1 -> MatrixSign_12_Conversion/1
  MatrixSign_12_Conversion/1 -> SubMuxMatrixSign/3

== system Demo_PreScanCarSim3D_ExtFMU_cs/HighwayOverhang_5/ENABLED/VISUMatrixSignLights_Mux ==
  MatrixSign_18 : Inport  Tag=inport/MatrixSign_18  PortDimensions=4  SampleTime=50/1000  BusOutputAsStruct=on
  MatrixSign_19 : Inport  Tag=inport/MatrixSign_19  Port=2  PortDimensions=4  SampleTime=50/1000  BusOutputAsStruct=on
  MatrixSign_20 : Inport  Tag=inport/MatrixSign_20  Port=3  PortDimensions=4  SampleTime=50/1000  BusOutputAsStruct=on
  MuxVisuLights : Mux  Inputs=3
  VISUMatrixSignLights_HighwayOverhang_5 : Outport  Tag=outport/VisuMatrixSignLights  SampleTime=50/1000
  wires:
  MuxVisuLights/1 -> VISUMatrixSignLights_HighwayOverhang_5/1
  MatrixSign_18/1 -> MuxVisuLights/1
  MatrixSign_19/1 -> MuxVisuLights/2
  MatrixSign_20/1 -> MuxVisuLights/3

== system Demo_PreScanCarSim3D_ExtFMU_cs/HighwayOverhang_5/ENABLED/VISUMatrixSign_Mux ==
  MatrixSign_18 : Inport
  MatrixSign_19 : Inport  Port=2
  MatrixSign_20 : Inport  Port=3
  MatrixSign_18_Conversion : DataTypeConversion
  MatrixSign_18_InitialResource : Constant  Value=11
  MatrixSign_18_Switch : Switch  Criteria=u2 ~= 0
  MatrixSign_19_Conversion : DataTypeConversion
  MatrixSign_19_InitialResource : Constant  Value=11
  MatrixSign_19_Switch : Switch  Criteria=u2 ~= 0
  MatrixSign_20_Conversion : DataTypeConversion
  MatrixSign_20_InitialResource : Constant  Value=11
  MatrixSign_20_Switch : Switch  Criteria=u2 ~= 0
  SubMuxMatrixSign : Mux  Inputs=3
  MatrixSigns : Outport
  wires:
  SubMuxMatrixSign/1 -> MatrixSigns/1
  MatrixSign_18/1 -> MatrixSign_18_Switch/1, MatrixSign_18_Switch/2
  MatrixSign_18_InitialResource/1 -> MatrixSign_18_Switch/3
  MatrixSign_18_Switch/1 -> MatrixSign_18_Conversion/1
  MatrixSign_18_Conversion/1 -> SubMuxMatrixSign/1
  MatrixSign_19/1 -> MatrixSign_19_Switch/1, MatrixSign_19_Switch/2
  MatrixSign_19_InitialResource/1 -> MatrixSign_19_Switch/3
  MatrixSign_19_Switch/1 -> MatrixSign_19_Conversion/1
  MatrixSign_19_Conversion/1 -> SubMuxMatrixSign/2
  MatrixSign_20/1 -> MatrixSign_20_Switch/1, MatrixSign_20_Switch/2
  MatrixSign_20_InitialResource/1 -> MatrixSign_20_Switch/3
  MatrixSign_20_Switch/1 -> MatrixSign_20_Conversion/1
  MatrixSign_20_Conversion/1 -> SubMuxMatrixSign/3

== system Demo_PreScanCarSim3D_ExtFMU_cs/SELF_Audi_A8_1/DISABLED/GND1 ==
  GND_Alt : Constant  Value=0
  GND_Lat : Constant  Value=0
  GND_Long : Constant  Value=0
  GND_OrientationPitch : Constant  Value=0
  GND_OrientationRoll : Constant  Value=0
  GND_OrientationYaw : Constant  Value=0
  GND_PositionX : Constant  Value=0
  GND_PositionY : Constant  Value=0
  GND_PositionZ : Constant  Value=0
  GND_Velocity : Constant  Value=0
  GND_Yaw_rate : Constant  Value=0
  buscreator : BusCreator  Inputs=11  OutDataTypeStr=Bus: PRESCAN_SELFSENSORDATA  NonVirtualBus=on
  bus : Outport  OutDataTypeStr=Bus: PRESCAN_SELFSENSORDATA
  wires:
  GND_PositionX/1 -> buscreator/1  "PositionX"
  GND_PositionY/1 -> buscreator/2  "PositionY"
  GND_PositionZ/1 -> buscreator/3  "PositionZ"
  GND_OrientationRoll/1 -> buscreator/4  "OrientationRoll"
  GND_OrientationPitch/1 -> buscreator/5  "OrientationPitch"
  GND_OrientationYaw/1 -> buscreator/6  "OrientationYaw"
  GND_Velocity/1 -> buscreator/7  "Velocity"
  GND_Yaw_rate/1 -> buscreator/8  "Yaw_rate"
  GND_Lat/1 -> buscreator/9  "Lat"
  GND_Long/1 -> buscreator/10  "Long"
  GND_Alt/1 -> buscreator/11  "Alt"
  buscreator/1 -> bus/1

== system Demo_PreScanCarSim3D_ExtFMU_cs/SELF_Box_1/DISABLED/GND1 ==
  GND_Alt : Constant  Value=0
  GND_Lat : Constant  Value=0
  GND_Long : Constant  Value=0
  GND_OrientationPitch : Constant  Value=0
  GND_OrientationRoll : Constant  Value=0
  GND_OrientationYaw : Constant  Value=0
  GND_PositionX : Constant  Value=0
  GND_PositionY : Constant  Value=0
  GND_PositionZ : Constant  Value=0
  GND_Velocity : Constant  Value=0
  GND_Yaw_rate : Constant  Value=0
  buscreator : BusCreator  Inputs=11  OutDataTypeStr=Bus: PRESCAN_SELFSENSORDATA  NonVirtualBus=on
  bus : Outport  OutDataTypeStr=Bus: PRESCAN_SELFSENSORDATA
  wires:
  GND_PositionX/1 -> buscreator/1  "PositionX"
  GND_PositionY/1 -> buscreator/2  "PositionY"
  GND_PositionZ/1 -> buscreator/3  "PositionZ"
  GND_OrientationRoll/1 -> buscreator/4  "OrientationRoll"
  GND_OrientationPitch/1 -> buscreator/5  "OrientationPitch"
  GND_OrientationYaw/1 -> buscreator/6  "OrientationYaw"
  GND_Velocity/1 -> buscreator/7  "Velocity"
  GND_Yaw_rate/1 -> buscreator/8  "Yaw_rate"
  GND_Lat/1 -> buscreator/9  "Lat"
  GND_Long/1 -> buscreator/10  "Long"
  GND_Alt/1 -> buscreator/11  "Alt"
  buscreator/1 -> bus/1

== system Demo_PreScanCarSim3D_ExtFMU_cs/SELF_Box_2/DISABLED/GND1 ==
  GND_Alt : Constant  Value=0
  GND_Lat : Constant  Value=0
  GND_Long : Constant  Value=0
  GND_OrientationPitch : Constant  Value=0
  GND_OrientationRoll : Constant  Value=0
  GND_OrientationYaw : Constant  Value=0
  GND_PositionX : Constant  Value=0
  GND_PositionY : Constant  Value=0
  GND_PositionZ : Constant  Value=0
  GND_Velocity : Constant  Value=0
  GND_Yaw_rate : Constant  Value=0
  buscreator : BusCreator  Inputs=11  OutDataTypeStr=Bus: PRESCAN_SELFSENSORDATA  NonVirtualBus=on
  bus : Outport  OutDataTypeStr=Bus: PRESCAN_SELFSENSORDATA
  wires:
  GND_PositionX/1 -> buscreator/1  "PositionX"
  GND_PositionY/1 -> buscreator/2  "PositionY"
  GND_PositionZ/1 -> buscreator/3  "PositionZ"
  GND_OrientationRoll/1 -> buscreator/4  "OrientationRoll"
  GND_OrientationPitch/1 -> buscreator/5  "OrientationPitch"
  GND_OrientationYaw/1 -> buscreator/6  "OrientationYaw"
  GND_Velocity/1 -> buscreator/7  "Velocity"
  GND_Yaw_rate/1 -> buscreator/8  "Yaw_rate"
  GND_Lat/1 -> buscreator/9  "Lat"
  GND_Long/1 -> buscreator/10  "Long"
  GND_Alt/1 -> buscreator/11  "Alt"
  buscreator/1 -> bus/1

== system Demo_PreScanCarSim3D_ExtFMU_cs/SELF_Box_3/DISABLED/GND1 ==
  GND_Alt : Constant  Value=0
  GND_Lat : Constant  Value=0
  GND_Long : Constant  Value=0
  GND_OrientationPitch : Constant  Value=0
  GND_OrientationRoll : Constant  Value=0
  GND_OrientationYaw : Constant  Value=0
  GND_PositionX : Constant  Value=0
  GND_PositionY : Constant  Value=0
  GND_PositionZ : Constant  Value=0
  GND_Velocity : Constant  Value=0
  GND_Yaw_rate : Constant  Value=0
  buscreator : BusCreator  Inputs=11  OutDataTypeStr=Bus: PRESCAN_SELFSENSORDATA  NonVirtualBus=on
  bus : Outport  OutDataTypeStr=Bus: PRESCAN_SELFSENSORDATA
  wires:
  GND_PositionX/1 -> buscreator/1  "PositionX"
  GND_PositionY/1 -> buscreator/2  "PositionY"
  GND_PositionZ/1 -> buscreator/3  "PositionZ"
  GND_OrientationRoll/1 -> buscreator/4  "OrientationRoll"
  GND_OrientationPitch/1 -> buscreator/5  "OrientationPitch"
  GND_OrientationYaw/1 -> buscreator/6  "OrientationYaw"
  GND_Velocity/1 -> buscreator/7  "Velocity"
  GND_Yaw_rate/1 -> buscreator/8  "Yaw_rate"
  GND_Lat/1 -> buscreator/9  "Lat"
  GND_Long/1 -> buscreator/10  "Long"
  GND_Alt/1 -> buscreator/11  "Alt"
  buscreator/1 -> bus/1

== system Demo_PreScanCarSim3D_ExtFMU_cs/SELF_Box_4/DISABLED/GND1 ==
  GND_Alt : Constant  Value=0
  GND_Lat : Constant  Value=0
  GND_Long : Constant  Value=0
  GND_OrientationPitch : Constant  Value=0
  GND_OrientationRoll : Constant  Value=0
  GND_OrientationYaw : Constant  Value=0
  GND_PositionX : Constant  Value=0
  GND_PositionY : Constant  Value=0
  GND_PositionZ : Constant  Value=0
  GND_Velocity : Constant  Value=0
  GND_Yaw_rate : Constant  Value=0
  buscreator : BusCreator  Inputs=11  OutDataTypeStr=Bus: PRESCAN_SELFSENSORDATA  NonVirtualBus=on
  bus : Outport  OutDataTypeStr=Bus: PRESCAN_SELFSENSORDATA
  wires:
  GND_PositionX/1 -> buscreator/1  "PositionX"
  GND_PositionY/1 -> buscreator/2  "PositionY"
  GND_PositionZ/1 -> buscreator/3  "PositionZ"
  GND_OrientationRoll/1 -> buscreator/4  "OrientationRoll"
  GND_OrientationPitch/1 -> buscreator/5  "OrientationPitch"
  GND_OrientationYaw/1 -> buscreator/6  "OrientationYaw"
  GND_Velocity/1 -> buscreator/7  "Velocity"
  GND_Yaw_rate/1 -> buscreator/8  "Yaw_rate"
  GND_Lat/1 -> buscreator/9  "Lat"
  GND_Long/1 -> buscreator/10  "Long"
  GND_Alt/1 -> buscreator/11  "Alt"
  buscreator/1 -> bus/1

== system Demo_PreScanCarSim3D_ExtFMU_cs/TrafficLightRoadSideNL_1/ENABLED/VISUCasingLights_Mux ==
  Green [-] : Inport  Tag=inport/Green [-]  SampleTime=50/1000  BusOutputAsStruct=on
  Orange [-] : Inport  Tag=inport/Orange [-]  Port=2  SampleTime=50/1000  BusOutputAsStruct=on
  Red [-] : Inport  Tag=inport/Red [-]  Port=3  SampleTime=50/1000  BusOutputAsStruct=on
  MuxVisuLights : Mux  Inputs=3
  VISUCasingLights_TrafficLightRoadSideNL_1 : Outport  Tag=outport/VisuCasingLights  SampleTime=50/1000
  wires:
  MuxVisuLights/1 -> VISUCasingLights_TrafficLightRoadSideNL_1/1
  Green [-]/1 -> MuxVisuLights/1
  Orange [-]/1 -> MuxVisuLights/2
  Red [-]/1 -> MuxVisuLights/3

== system Demo_PreScanCarSim3D_ExtFMU_cs/TrafficLightRoadSideNL_2/ENABLED/VISUCasingLights_Mux ==
  Green [-] : Inport  Tag=inport/Green [-]  SampleTime=50/1000  BusOutputAsStruct=on
  Orange [-] : Inport  Tag=inport/Orange [-]  Port=2  SampleTime=50/1000  BusOutputAsStruct=on
  Red [-] : Inport  Tag=inport/Red [-]  Port=3  SampleTime=50/1000  BusOutputAsStruct=on
  MuxVisuLights : Mux  Inputs=3
  VISUCasingLights_TrafficLightRoadSideNL_2 : Outport  Tag=outport/VisuCasingLights  SampleTime=50/1000
  wires:
  MuxVisuLights/1 -> VISUCasingLights_TrafficLightRoadSideNL_2/1
  Green [-]/1 -> MuxVisuLights/1
  Orange [-]/1 -> MuxVisuLights/2
  Red [-]/1 -> MuxVisuLights/3

== system Demo_PreScanCarSim3D_ExtFMU_cs/TrafficLightRoadSideNL_3/ENABLED/VISUCasingLights_Mux ==
  Green [-] : Inport  Tag=inport/Green [-]  SampleTime=50/1000  BusOutputAsStruct=on
  Orange [-] : Inport  Tag=inport/Orange [-]  Port=2  SampleTime=50/1000  BusOutputAsStruct=on
  Red [-] : Inport  Tag=inport/Red [-]  Port=3  SampleTime=50/1000  BusOutputAsStruct=on
  MuxVisuLights : Mux  Inputs=3
  VISUCasingLights_TrafficLightRoadSideNL_3 : Outport  Tag=outport/VisuCasingLights  SampleTime=50/1000
  wires:
  MuxVisuLights/1 -> VISUCasingLights_TrafficLightRoadSideNL_3/1
  Green [-]/1 -> MuxVisuLights/1
  Orange [-]/1 -> MuxVisuLights/2
  Red [-]/1 -> MuxVisuLights/3

== system Demo_PreScanCarSim3D_ExtFMU_cs/TrafficLightRoadSideNL_5/ENABLED/VISUCasingLights_Mux ==
  Green [-] : Inport  Tag=inport/Green [-]  SampleTime=50/1000  BusOutputAsStruct=on
  Orange [-] : Inport  Tag=inport/Orange [-]  Port=2  SampleTime=50/1000  BusOutputAsStruct=on
  Red [-] : Inport  Tag=inport/Red [-]  Port=3  SampleTime=50/1000  BusOutputAsStruct=on
  MuxVisuLights : Mux  Inputs=3
  VISUCasingLights_TrafficLightRoadSideNL_5 : Outport  Tag=outport/VisuCasingLights  SampleTime=50/1000
  wires:
  MuxVisuLights/1 -> VISUCasingLights_TrafficLightRoadSideNL_5/1
  Green [-]/1 -> MuxVisuLights/1
  Orange [-]/1 -> MuxVisuLights/2
  Red [-]/1 -> MuxVisuLights/3

== system Demo_PreScanCarSim3D_ExtFMU_cs/TrafficLightRoadSideNL_6/ENABLED/VISUCasingLights_Mux ==
  Green [-] : Inport  Tag=inport/Green [-]  SampleTime=50/1000  BusOutputAsStruct=on
  Orange [-] : Inport  Tag=inport/Orange [-]  Port=2  SampleTime=50/1000  BusOutputAsStruct=on
  Red [-] : Inport  Tag=inport/Red [-]  Port=3  SampleTime=50/1000  BusOutputAsStruct=on
  MuxVisuLights : Mux  Inputs=3
  VISUCasingLights_TrafficLightRoadSideNL_6 : Outport  Tag=outport/VisuCasingLights  SampleTime=50/1000
  wires:
  MuxVisuLights/1 -> VISUCasingLights_TrafficLightRoadSideNL_6/1
  Green [-]/1 -> MuxVisuLights/1
  Orange [-]/1 -> MuxVisuLights/2
  Red [-]/1 -> MuxVisuLights/3

== system Demo_PreScanCarSim3D_ExtFMU_cs/TrafficLightRoadSideNL_7/ENABLED/VISUCasingLights_Mux ==
  Green [-] : Inport  Tag=inport/Green [-]  SampleTime=50/1000  BusOutputAsStruct=on
  Orange [-] : Inport  Tag=inport/Orange [-]  Port=2  SampleTime=50/1000  BusOutputAsStruct=on
  Red [-] : Inport  Tag=inport/Red [-]  Port=3  SampleTime=50/1000  BusOutputAsStruct=on
  MuxVisuLights : Mux  Inputs=3
  VISUCasingLights_TrafficLightRoadSideNL_7 : Outport  Tag=outport/VisuCasingLights  SampleTime=50/1000
  wires:
  MuxVisuLights/1 -> VISUCasingLights_TrafficLightRoadSideNL_7/1
  Green [-]/1 -> MuxVisuLights/1
  Orange [-]/1 -> MuxVisuLights/2
  Red [-]/1 -> MuxVisuLights/3
